simulink model "LotkaVoterra"  (Simulink 6.6)
settings: Solver=ode45  StartTime=0.0  StopTime=10  RelTol=1e-3
settings Model: Creator=MXKana  LastModifiedBy=mxkana

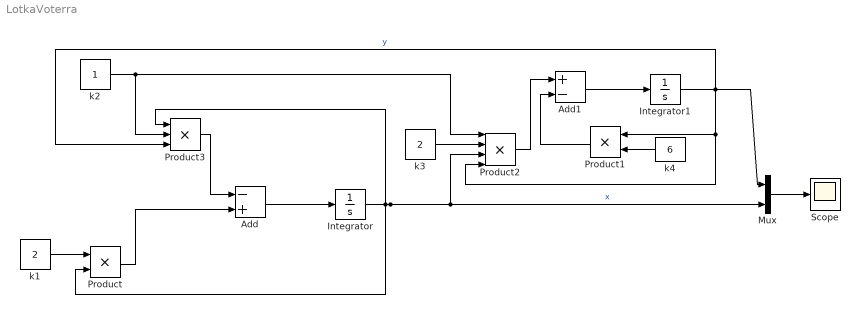
== system LotkaVoterra ==
  Add : Sum  Inputs=-+  OutScaling=2^-10
  Add1 : Sum  Inputs=+-  OutScaling=2^-10
  Integrator : Integrator  InitialCondition=1
  Integrator1 : Integrator  InitialCondition=1
  Mux : Mux  Inputs=2
  Product : Product  RndMeth=Zero
  Product1 : Product  Orientation=left  RndMeth=Zero
  Product2 : Product  Inputs=4  RndMeth=Zero
  Product3 : Product  Inputs=3  RndMeth=Zero
  Scope : Scope
  k1 : Constant  Value=2
  k2 : Constant
  k3 : Constant  Value=2
  k4 : Constant  Orientation=left  Value=6
  wires:
  Product/1 -> Add/2
  k1/1 -> Product/1
  Integrator/1 -> Product2/3, Mux/2, Product/2, Product3/1  "x"
  Add1/1 -> Integrator1/1
  Mux/1 -> Scope/1
  k2/1 -> Product2/1, Product3/2
  k3/1 -> Product2/2
  Product2/1 -> Add1/1
  Integrator1/1 -> Product3/3, Product2/4, Product1/1, Mux/1  "y"
  Add/1 -> Integrator/1
  Product3/1 -> Add/1
  k4/1 -> Product1/2
  Product1/1 -> Add1/2
